simulink model "q_5"  (R2020a)
settings: Solver=VariableStepAuto  StartTime=0.0  StopTime=10.0  RelTol=1e-3
values from neighbouring files (symbols this model uses):
  C = 1e-06    [rlc.mat]
  R = 10    [rlc.mat]
settings Model: EnablePacing=on  PacingRate=3  Creator=Admin  LastModifiedBy=Admin

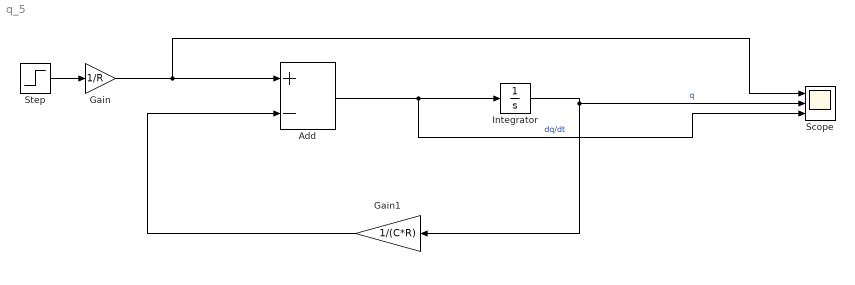
== system q_5 ==
  Add : Sum  Inputs=+-
  Gain : Gain  Gain=1/R
  Gain1 : Gain  Gain=1/(C*R)
  Integrator : Integrator
  Scope : Scope  NumInputPorts=3
  Step : Step  SampleTime=0
  wires:
  Add/1 -> Scope/3, Integrator/1  "dq/dt"
  Integrator/1 -> Gain1/1, Scope/2  "q"
  Gain/1 -> Scope/1, Add/1
  Gain1/1 -> Add/2
  Step/1 -> Gain/1
